simulink model "MinCylinderTester"  (R2015a)
settings: Solver=ode45  StartTime=0.0  StopTime=10.0  RelTol=1e-3
settings Model: Creator=user  LastModifiedBy=user

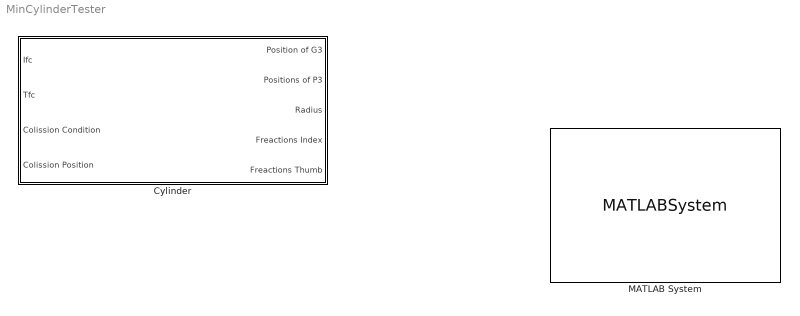
== system MinCylinderTester ==
  Cylinder : Subsystem
  MATLAB System : MATLABSystem  System=MinCylinderTester  R=[]  M=[]  g=[]  Us=[]  Uk=[]  Urs=[]  Urk=[]  Ucs=[]  Uck=[]  Iz=[]  F_s_x=[]  F_s_y=[]  F_k_x=[]  F_k_y=[]  T_s=[]  T_k=[]  Position_o_G3=[]  Position_G3_P3_frame_cylinder=[ 0; 0 ]  SimulateUsing=Code generation
      mask Type: MinCylinderTester
      mask Display:
      | disp('MinCylinderTester');
      | port_label('input',1,'Urk');
      | port_label('input',2,'IndexFext');
      | port_label('input',3,'ThumbFext');
      | port_label('input',4,'CollisionCondition');
      | port_label('input',5,'CollisionPosition');
      | port_label('input',6,'xDotG3');
      | port_label('input',7,'yDotG3');
      | port_label('input',8,'angleDot');
      | port_label('input',9,'xPositionG3');
      | port_label('input',10,'yPositionG3');
      | port_label('input',11,'angle');
      | port_label('output',1,'CylinderResults');

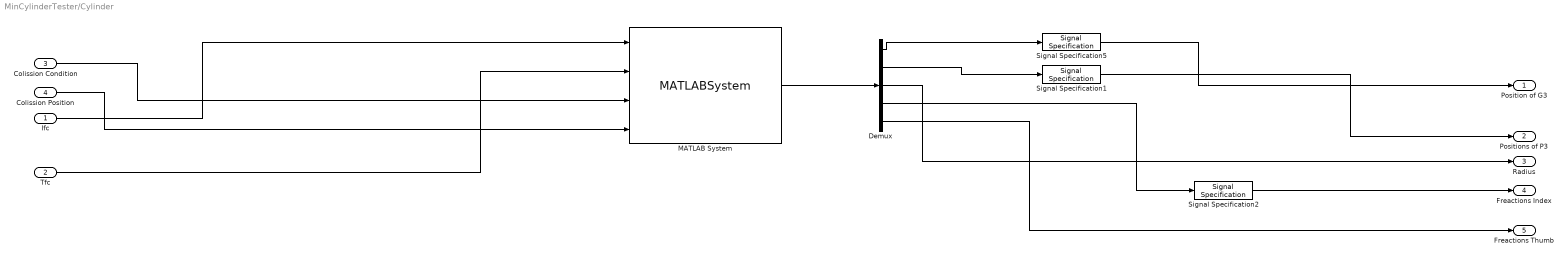
== system MinCylinderTester/Cylinder ==
  Ifc : Inport
  Tfc : Inport  Port=2
  Colission Condition : Inport  Port=3
  Colission Position : Inport  Port=4
  Demux : Demux  Outputs=5
  MATLAB System : MATLABSystem  System=MinCylinderTester  R=[]  M=[]  g=[]  Us=[]  Uk=[]  Urs=[]  Urk=[]  Ucs=[]  Uck=[]  Iz=[]  F_s_x=[]  F_s_y=[]  F_k_x=[]  F_k_y=[]  T_s=[]  T_k=[]  Position_o_G3=[]  Position_G3_P3_frame_cylinder=[ 0; 0 ]  SimulateUsing=Code generation
      mask Type: MinCylinderTester
      mask Display:
      | disp('MinCylinderTester');
      | port_label('input',1,'IndexFext');
      | port_label('input',2,'ThumbFext');
      | port_label('input',3,'CollisionCondition');
      | port_label('input',4,'CollisionPosition');
      | port_label('output',1,'CylinderResults');
  Signal Specification1 : SignalSpecification  Dimensions=2
  Signal Specification2 : SignalSpecification  Dimensions=2
  Signal Specification5 : SignalSpecification  Dimensions=2
  " Position of G3" : Outport
  Positions of P3 : Outport  Port=2
  Radius : Outport  Port=3
  Freactions Index : Outport  Port=4
  Freactions Thumb : Outport  Port=5
  wires:
  Colission Condition/1 -> MATLAB System/3
  Colission Position/1 -> MATLAB System/4
  Ifc/1 -> MATLAB System/1
  Tfc/1 -> MATLAB System/2
  MATLAB System/1 -> Demux/1
  Demux/1 -> Signal Specification5/1
  Signal Specification5/1 -> " Position of G3"/1
  Demux/2 -> Signal Specification1/1
  Signal Specification1/1 -> Positions of P3/1
  Demux/3 -> Radius/1
  Demux/4 -> Signal Specification2/1
  Signal Specification2/1 -> Freactions Index/1
  Demux/5 -> Freactions Thumb/1
